simulink model "SkywalkerX8_Longitudinal_Control_Digital_Verification"  (R2018a)
settings: Solver=FixedStepAuto  StartTime=0.0  StopTime=10  RelTol=1e-3
undefined symbols (not defined in the file): DiscIntNeverNeededParam, SkywalkerX8
libraries: simulink_extras x5, simulink x1
settings Model: SnapshotInterval=1  Creator=David  LastModifiedBy=David
settings SolverCC: AlgebraicLoopSolver=LineSearch

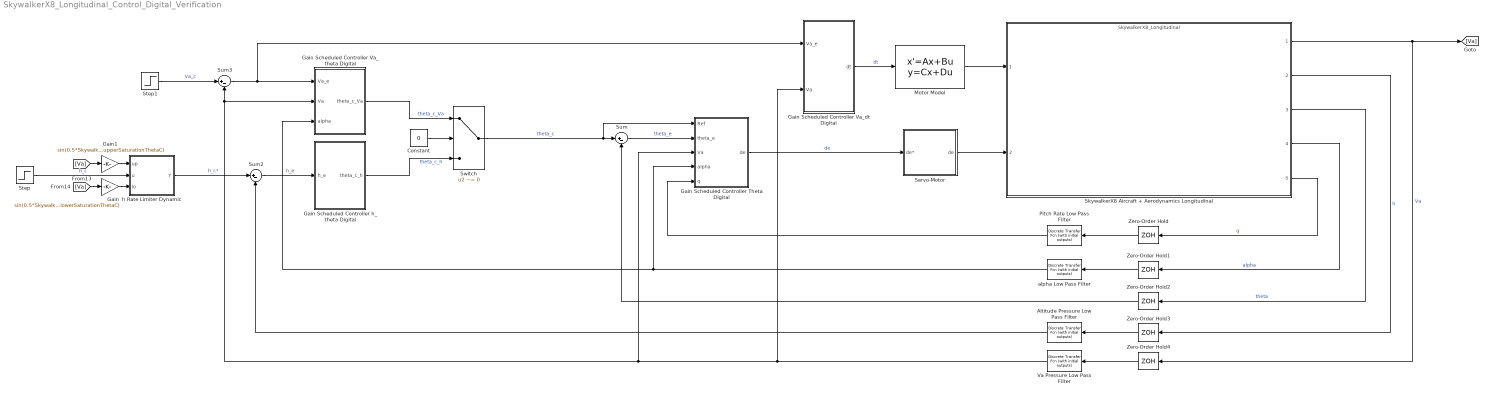
== system SkywalkerX8_Longitudinal_Control_Digital_Verification ==
  Altitude Pressure Low Pass Filter : simulink_extras/Additional Discrete/Discrete Transfer Fcn (with initial outputs)  N=cell2mat(SkywalkerX8.Sensors.Filters.AltitudePressure.FilterTFDigital.Numerator)  D=cell2mat(SkywalkerX8.Sensors.Filters.AltitudePressure.FilterTFDigital.Denominator)  U0=-SkywalkerX8.InitialConditions.XeYeZe(3)  Y0=-SkywalkerX8.InitialConditions.XeYeZe(3)  TS=SkywalkerX8.Sensors.Filters.AltitudePressure.FilterSampleTime
      settings: SourceProductName=Simulink  SourceProductBaseCode=SL
  Constant : Constant  Value=0  OutDataTypeStr=boolean
  Gain : Gain  Gain=sin(0.5*SkywalkerX8.Control.Longitudinal.altController.lowerSaturationThetaC)
  Gain Scheduled Controller Theta Digital : Subsystem
  Gain Scheduled Controller Va_dt Digital : Subsystem
  Gain Scheduled Controller Va_theta Digital : Subsystem
  Gain Scheduled Controller h_theta Digital : Subsystem
  Gain1 : Gain  Gain=sin(0.5*SkywalkerX8.Control.Longitudinal.altController.upperSaturationThetaC)
  Motor Model : StateSpace  A=SkywalkerX8.Actuators.Motor.SS.A  B=SkywalkerX8.Actuators.Motor.SS.B  C=SkywalkerX8.Actuators.Motor.SS.C  D=SkywalkerX8.Actuators.Motor.SS.D  InitialCondition=SkywalkerX8.InitialConditions.dt/SkywalkerX8.Actuators.Motor.SS.C
      mask Display: image('motor.jpg', 'center')
  Pitch Rate Low Pass Filter : simulink_extras/Additional Discrete/Discrete Transfer Fcn (with initial outputs)  N=cell2mat(SkywalkerX8.Sensors.Filters.AngularRates.Pitch.FilterTFDigital.Numerator)  D=cell2mat(SkywalkerX8.Sensors.Filters.AngularRates.Pitch.FilterTFDigital.Denominator)  U0=SkywalkerX8.Sensors.Filters.AngularRates.Pitch.InitialCondition  Y0=SkywalkerX8.Sensors.Filters.AngularRates.Pitch.InitialCondition  TS=SkywalkerX8.Sensors.Filters.AngularRates.Pitch.FilterSampleTime
      settings: SourceProductName=Simulink  SourceProductBaseCode=SL
  Servo-Motor : Subsystem
      mask Display: image('servo.jpg', 'center')
  SkywalkerX8 Aircraft + Aerodynamics Longitudinal : ModelReference  ModelNameDialog=SkywalkerX8_Longitudinal  ModelReferenceVersion=1.65
      mask Display:
      | image('x8SkySunset.png', 'center')
      | 
      | port_label('input', 1, '\delta_t (Unitless)', 'texmode', 'on')
      | port_label('input', 2, '\delta_e (rad)', 'texmode', 'on')
      | 
      | port_label('output', 1, 'V_a (m/s)', 'texmode', 'on')
      | port_label('output', 2, 'Altitude (m)', 'texmode', 'on')
      | port_label('output', 3, '\theta (rad)', 'texmode', 'on')
      | port_label('output', 4, 'alpha (rad)', 'texmode', 'on')
      | port_label('output', 5, 'q (rad/s)', 'texmode', 'on')
  Step : Step  Time=0.1  Before=-SkywalkerX8.InitialConditions.XeYeZe(3)  After=-SkywalkerX8.InitialConditions.XeYeZe(3)  SampleTime=0
  Step1 : Step  Time=5  Before=sqrt(SkywalkerX8.InitialConditions.uvw*SkywalkerX8.InitialConditions.uvw')  After=1.25*sqrt(SkywalkerX8.InitialConditions.uvw*SkywalkerX8.InitialConditions.uvw')  SampleTime=0
  Sum : Sum  Inputs=|+-
  Sum2 : Sum  Inputs=|+-
  Sum3 : Sum  Inputs=|+-
  Switch : Switch  Criteria=u2 ~= 0
  Va Pressure Low Pass Filter : simulink_extras/Additional Discrete/Discrete Transfer Fcn (with initial outputs)  N=cell2mat(SkywalkerX8.Sensors.Filters.AirspeedPressure.FilterTFDigital.Numerator)  D=cell2mat(SkywalkerX8.Sensors.Filters.AirspeedPressure.FilterTFDigital.Denominator)  U0=sqrt(SkywalkerX8.InitialConditions.uvw*SkywalkerX8.InitialConditions.uvw')  Y0=sqrt(SkywalkerX8.InitialConditions.uvw*SkywalkerX8.InitialConditions.uvw')  TS=SkywalkerX8.Sensors.Filters.AirspeedPressure.FilterSampleTime
      settings: SourceProductName=Simulink  SourceProductBaseCode=SL
  Zero-Order Hold : ZeroOrderHold  SampleTime=SkywalkerX8.Sensors.IMU.Gyroscope.SampleTime
  Zero-Order Hold1 : ZeroOrderHold  SampleTime=SkywalkerX8.Sensors.AoA.SampleTime
  Zero-Order Hold2 : ZeroOrderHold  SampleTime=SkywalkerX8.Sensors.EKF.GPSSmoothing.StateTransitionSampleTime
  Zero-Order Hold3 : ZeroOrderHold  SampleTime=SkywalkerX8.Sensors.AltitudePressure.SampleTime
  Zero-Order Hold4 : ZeroOrderHold  SampleTime=SkywalkerX8.Sensors.AirspeedPressure.SampleTime
  alpha Low Pass Filter : simulink_extras/Additional Discrete/Discrete Transfer Fcn (with initial outputs)  N=cell2mat(SkywalkerX8.Sensors.Filters.AoA.FilterTFDigital.Numerator)  D=cell2mat(SkywalkerX8.Sensors.Filters.AoA.FilterTFDigital.Denominator)  U0=SkywalkerX8.Sensors.Filters.AoA.InitialCondition  Y0=SkywalkerX8.Sensors.Filters.AoA.InitialCondition  TS=SkywalkerX8.Sensors.Filters.AoA.FilterSampleTime
      settings: SourceProductName=Simulink  SourceProductBaseCode=SL
  h Rate Limiter Dynamic : Subsystem  mask{initOutput=-SkywalkerX8.InitialConditions.XeYeZe(3)}
      mask prompts: initOutput "Initial output of dynamic rate limiter"
      mask DialogControl DescGroupVar Prompt: Rate Limiter Dynamic
      mask DialogControl DescTextVar Prompt: Limit rising and falling rates of the signals at the second input by using the first input (upper limit) and the third input (lower limit).
      mask Display:
      | image('rateLimit.png')
      | 
      | port_label('input', 1, 'up')
      | port_label('input', 2, 'u')
      | port_label('input', 3, 'lo')
      | 
      | port_label('output', 1, 'Y')
  wires:
  SkywalkerX8 Aircraft + Aerodynamics Longitudinal/5 -> Zero-Order Hold/1  "q"
  SkywalkerX8 Aircraft + Aerodynamics Longitudinal/3 -> Zero-Order Hold2/1  "theta"
  Constant/1 -> Switch/2
  SkywalkerX8 Aircraft + Aerodynamics Longitudinal/2 -> Zero-Order Hold3/1  "h"
  Sum2/1 -> Gain Scheduled Controller h_theta Digital/1(h_e)  "h_e"
  SkywalkerX8 Aircraft + Aerodynamics Longitudinal/1 -> Zero-Order Hold4/1, [Va]  "Va"
  Gain Scheduled Controller Va_theta Digital/1(theta_c_Va) -> Switch/1  "theta_c_Va"
  Step1/1 -> Sum3/1  "Va_c"
  Sum/1 -> Gain Scheduled Controller Theta Digital/2(theta_e)  "theta_e"
  SkywalkerX8 Aircraft + Aerodynamics Longitudinal/4 -> Zero-Order Hold1/1  "alpha"
  Gain Scheduled Controller h_theta Digital/1(theta_c_h) -> Switch/3  "theta_c_h"
  Gain Scheduled Controller Va_dt Digital/1(dt) -> Motor Model/1  "dt"
  h Rate Limiter Dynamic/1(Y) -> Sum2/1  "h_c*"
  Gain Scheduled Controller Theta Digital/1(de) -> Servo-Motor/1(de*)  "de"
  Sum3/1 -> Gain Scheduled Controller Va_theta Digital/1(Va_e), Gain Scheduled Controller Va_dt Digital/1(Va_e)
  Zero-Order Hold1/1 -> alpha Low Pass Filter/1
  Zero-Order Hold3/1 -> Altitude Pressure Low Pass Filter/1
  Zero-Order Hold4/1 -> Va Pressure Low Pass Filter/1
  Motor Model/1 -> SkywalkerX8 Aircraft + Aerodynamics Longitudinal/1
  Servo-Motor/1(de) -> SkywalkerX8 Aircraft + Aerodynamics Longitudinal/2
  Switch/1 -> Gain Scheduled Controller Theta Digital/1(Ref), Sum/1  "theta_c"
  Gain/1 -> h Rate Limiter Dynamic/3(lo)
  [Va] -> Gain1/1
  Gain1/1 -> h Rate Limiter Dynamic/1(up)
  [Va] -> Gain/1
  Step/1 -> h Rate Limiter Dynamic/2(u)  "h_c"
  Zero-Order Hold2/1 -> Sum/2
  Zero-Order Hold/1 -> Pitch Rate Low Pass Filter/1
  Altitude Pressure Low Pass Filter/1 -> Sum2/2
  Va Pressure Low Pass Filter/1 -> Gain Scheduled Controller Va_theta Digital/2(Va), Sum3/2, Gain Scheduled Controller Theta Digital/3(Va), Gain Scheduled Controller Va_dt Digital/2(Va)
  Pitch Rate Low Pass Filter/1 -> Gain Scheduled Controller Theta Digital/5(q)
  alpha Low Pass Filter/1 -> Gain Scheduled Controller Theta Digital/4(alpha), Gain Scheduled Controller Va_theta Digital/3(alpha)

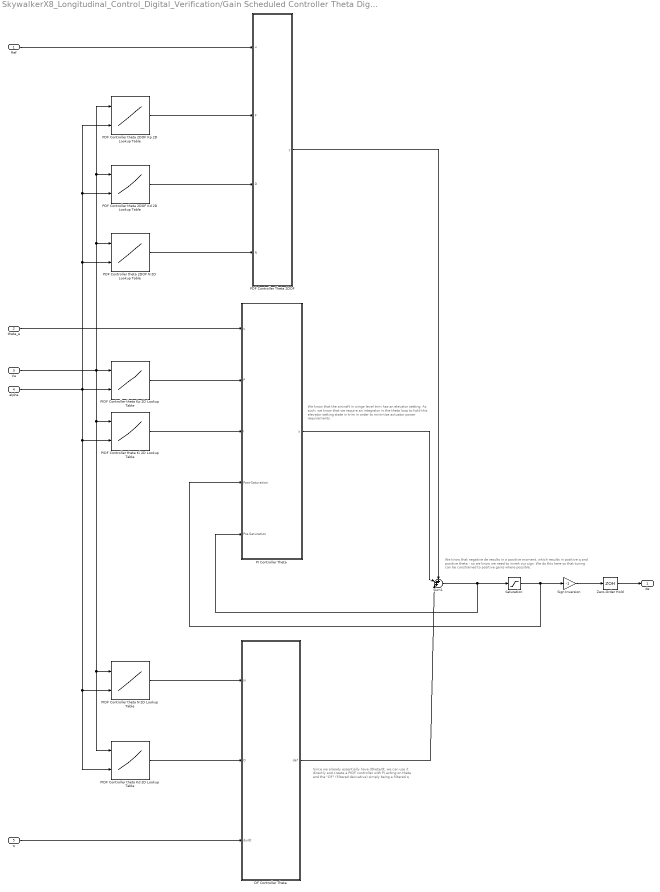
== system SkywalkerX8_Longitudinal_Control_Digital_Verification/Gain Scheduled Controller Theta Digital ==
  note: Since we already essentially have dtheta/dt,
      | we can use it directly and create a PIDF controller
      | with PI acting on theta and the "DF" (filtered derivative)
      | simply being a filtered q
  note: We know that negative de results in a positive moment, which results in
      | positive q and positive theta - so we know we need to invert our sign.
      | We do this here so that tuning can be constrained to positive gains where possible.
  note: We know that the aircraft in wings-level trim has an elevator setting. As such, we know that we require an integrator in the theta loop to hold this elevator setting state in trim in order to minimize actuator power requirements.
  Ref : Inport
  theta_e : Inport  Port=2
  Va : Inport  Port=3
  alpha : Inport  Port=4
  q : Inport  Port=5
  DF Controller Theta : Subsystem
  PDF Controller Theta 2DOF : Subsystem
  PDF Controller theta 2DOF Kd 2D Lookup Table : Lookup_n-D  BreakpointsForDimension1=SkywalkerX8.Control.Longitudinal.SchedulingVariables.VaArray  BreakpointsForDimension2=SkywalkerX8.Control.Longitudinal.SchedulingVariables.alphaArray  Table=SkywalkerX8.Control.Longitudinal.thetaController.Digital.KdTheta2DOF  InternalRulePriority=Speed  RndMeth=Simplest  InputSameDT=on
  PDF Controller theta 2DOF Kp 2D Lookup Table : Lookup_n-D  BreakpointsForDimension1=SkywalkerX8.Control.Longitudinal.SchedulingVariables.VaArray  BreakpointsForDimension2=SkywalkerX8.Control.Longitudinal.SchedulingVariables.alphaArray  Table=SkywalkerX8.Control.Longitudinal.thetaController.Digital.KpTheta2DOF  InternalRulePriority=Speed  RndMeth=Simplest  InputSameDT=on
  PDF Controller theta 2DOF N 2D Lookup Table : Lookup_n-D  BreakpointsForDimension1=SkywalkerX8.Control.Longitudinal.SchedulingVariables.VaArray  BreakpointsForDimension2=SkywalkerX8.Control.Longitudinal.SchedulingVariables.alphaArray  Table=SkywalkerX8.Control.Longitudinal.thetaController.Digital.NTheta2DOF  InternalRulePriority=Speed  RndMeth=Simplest  InputSameDT=on
  PI Controller Theta : Subsystem
  PIDF Controller theta Kd 2D Lookup Table : Lookup_n-D  BreakpointsForDimension1=SkywalkerX8.Control.Longitudinal.SchedulingVariables.VaArray  BreakpointsForDimension2=SkywalkerX8.Control.Longitudinal.SchedulingVariables.alphaArray  Table=SkywalkerX8.Control.Longitudinal.thetaController.Digital.KdTheta  InternalRulePriority=Speed  RndMeth=Simplest  InputSameDT=on
  PIDF Controller theta Ki 2D Lookup Table : Lookup_n-D  BreakpointsForDimension1=SkywalkerX8.Control.Longitudinal.SchedulingVariables.VaArray  BreakpointsForDimension2=SkywalkerX8.Control.Longitudinal.SchedulingVariables.alphaArray  Table=SkywalkerX8.Control.Longitudinal.thetaController.Digital.KiTheta  InternalRulePriority=Speed  RndMeth=Simplest  InputSameDT=on
  PIDF Controller theta Kp 2D Lookup Table : Lookup_n-D  BreakpointsForDimension1=SkywalkerX8.Control.Longitudinal.SchedulingVariables.VaArray  BreakpointsForDimension2=SkywalkerX8.Control.Longitudinal.SchedulingVariables.alphaArray  Table=SkywalkerX8.Control.Longitudinal.thetaController.Digital.KpTheta  InternalRulePriority=Speed  RndMeth=Simplest  InputSameDT=on
  PIDF Controller theta N 2D Lookup Table : Lookup_n-D  BreakpointsForDimension1=SkywalkerX8.Control.Longitudinal.SchedulingVariables.VaArray  BreakpointsForDimension2=SkywalkerX8.Control.Longitudinal.SchedulingVariables.alphaArray  Table=SkywalkerX8.Control.Longitudinal.thetaController.Digital.NTheta  InternalRulePriority=Speed  RndMeth=Simplest  InputSameDT=on
  Saturation : Saturate  UpperLimit=SkywalkerX8.Control.Longitudinal.thetaController.Digital.upperSaturationNegativeDe  LowerLimit=SkywalkerX8.Control.Longitudinal.thetaController.Digital.lowerSaturationNegativeDe
  Sign Inversion : Gain  Gain=-1
  Sum1 : Sum  Inputs=+++|
  Zero-Order Hold : ZeroOrderHold  SampleTime=SkywalkerX8.Control.Longitudinal.thetaController.Digital.SampleTime
  de : Outport
  wires:
  Va/1 -> PDF Controller theta 2DOF Kd 2D Lookup Table/1, PDF Controller theta 2DOF Kp 2D Lookup Table/1, PDF Controller theta 2DOF N 2D Lookup Table/1, PIDF Controller theta N 2D Lookup Table/1, PIDF Controller theta Kd 2D Lookup Table/1, PIDF Controller theta Ki 2D Lookup Table/1, PIDF Controller theta Kp 2D Lookup Table/1
  theta_e/1 -> PI Controller Theta/1(u)
  PIDF Controller theta Kp 2D Lookup Table/1 -> PI Controller Theta/2(P)
  PIDF Controller theta Ki 2D Lookup Table/1 -> PI Controller Theta/3(I)
  alpha/1 -> PDF Controller theta 2DOF N 2D Lookup Table/2, PDF Controller theta 2DOF Kd 2D Lookup Table/2, PDF Controller theta 2DOF Kp 2D Lookup Table/2, PIDF Controller theta N 2D Lookup Table/2, PIDF Controller theta Kd 2D Lookup Table/2, PIDF Controller theta Ki 2D Lookup Table/2, PIDF Controller theta Kp 2D Lookup Table/2
  PI Controller Theta/1(y) -> Sum1/2
  Sum1/1 -> Saturation/1, PI Controller Theta/5(Pre-Saturation)
  Saturation/1 -> Sign Inversion/1, PI Controller Theta/4(Post-Saturation)
  PIDF Controller theta N 2D Lookup Table/1 -> DF Controller Theta/1(N)
  PIDF Controller theta Kd 2D Lookup Table/1 -> DF Controller Theta/2(D)
  q/1 -> DF Controller Theta/3(du/dt)
  DF Controller Theta/1(de*) -> Sum1/3
  Sign Inversion/1 -> Zero-Order Hold/1
  PDF Controller theta 2DOF Kp 2D Lookup Table/1 -> PDF Controller Theta 2DOF/2(P)
  PDF Controller theta 2DOF Kd 2D Lookup Table/1 -> PDF Controller Theta 2DOF/3(D)
  PDF Controller theta 2DOF N 2D Lookup Table/1 -> PDF Controller Theta 2DOF/4(N)
  Ref/1 -> PDF Controller Theta 2DOF/1(u)
  PDF Controller Theta 2DOF/1(y) -> Sum1/1
  Zero-Order Hold/1 -> de/1

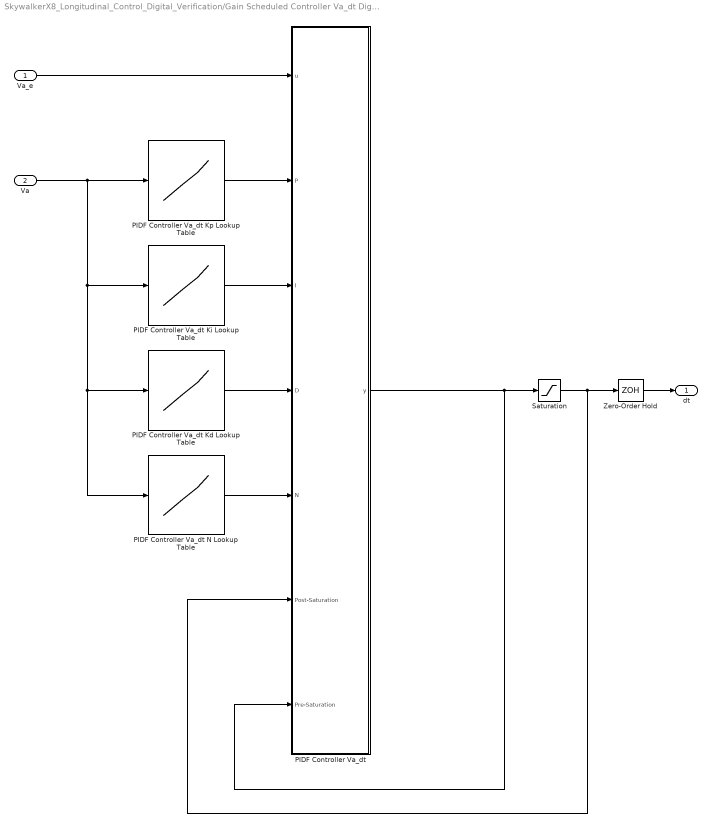
== system SkywalkerX8_Longitudinal_Control_Digital_Verification/Gain Scheduled Controller Va_dt Digital ==
  Va_e : Inport
  Va : Inport  Port=2
  PIDF Controller Va_dt : Subsystem
  PIDF Controller Va_dt Kd Lookup Table : Lookup_n-D  NumberOfTableDimensions=1  BreakpointsForDimension1=SkywalkerX8.Control.Longitudinal.SchedulingVariables.VaArray  BreakpointsForDimension2=[1 2 3 4 5]  Table=SkywalkerX8.Control.Longitudinal.VaDtController.Digital.KdVaDt  InternalRulePriority=Speed  RndMeth=Simplest  InputSameDT=on
  PIDF Controller Va_dt Ki Lookup Table : Lookup_n-D  NumberOfTableDimensions=1  BreakpointsForDimension1=SkywalkerX8.Control.Longitudinal.SchedulingVariables.VaArray  BreakpointsForDimension2=[1 2 3 4 5]  Table=SkywalkerX8.Control.Longitudinal.VaDtController.Digital.KiVaDt  InternalRulePriority=Speed  RndMeth=Simplest  InputSameDT=on
  PIDF Controller Va_dt Kp Lookup Table : Lookup_n-D  NumberOfTableDimensions=1  BreakpointsForDimension1=SkywalkerX8.Control.Longitudinal.SchedulingVariables.VaArray  BreakpointsForDimension2=[1 2 3 4 5]  Table=SkywalkerX8.Control.Longitudinal.VaDtController.Digital.KpVaDt  InternalRulePriority=Speed  RndMeth=Simplest  InputSameDT=on
  PIDF Controller Va_dt N Lookup Table : Lookup_n-D  NumberOfTableDimensions=1  BreakpointsForDimension1=SkywalkerX8.Control.Longitudinal.SchedulingVariables.VaArray  BreakpointsForDimension2=[1 2 3 4 5]  Table=SkywalkerX8.Control.Longitudinal.VaDtController.Digital.NVaDt  InternalRulePriority=Speed  RndMeth=Simplest  InputSameDT=on
  Saturation : Saturate  UpperLimit=SkywalkerX8.Control.Longitudinal.VaDtController.upperSaturationDt  LowerLimit=SkywalkerX8.Control.Longitudinal.VaDtController.lowerSaturationDt
  Zero-Order Hold : ZeroOrderHold  SampleTime=SkywalkerX8.Control.Longitudinal.VaDtController.Digital.SampleTime
  dt : Outport
  wires:
  Va_e/1 -> PIDF Controller Va_dt/1(u)
  Saturation/1 -> PIDF Controller Va_dt/6(Post-Saturation), Zero-Order Hold/1
  PIDF Controller Va_dt Kp Lookup Table/1 -> PIDF Controller Va_dt/2(P)
  Va/1 -> PIDF Controller Va_dt Kp Lookup Table/1, PIDF Controller Va_dt N Lookup Table/1, PIDF Controller Va_dt Kd Lookup Table/1, PIDF Controller Va_dt Ki Lookup Table/1
  PIDF Controller Va_dt Ki Lookup Table/1 -> PIDF Controller Va_dt/3(I)
  PIDF Controller Va_dt Kd Lookup Table/1 -> PIDF Controller Va_dt/4(D)
  PIDF Controller Va_dt N Lookup Table/1 -> PIDF Controller Va_dt/5(N)
  PIDF Controller Va_dt/1(y) -> Saturation/1, PIDF Controller Va_dt/7(Pre-Saturation)
  Zero-Order Hold/1 -> dt/1

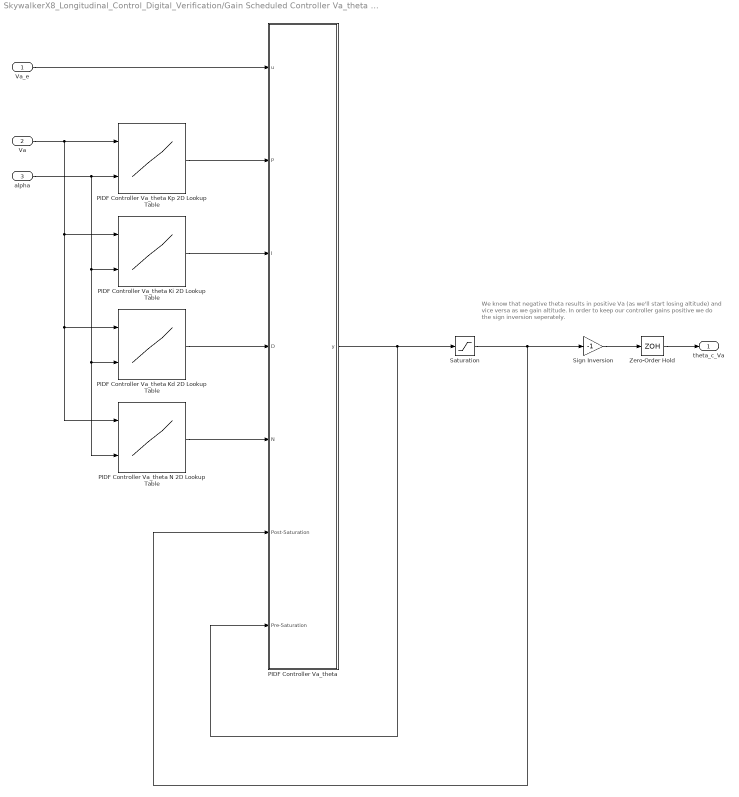
== system SkywalkerX8_Longitudinal_Control_Digital_Verification/Gain Scheduled Controller Va_theta Digital ==
  note: We know that negative theta results in positive Va (as we'll start losing altitude)
      | and vice versa as we gain altitude. In order to keep our controller gains positive
      |  we do the sign inversion seperately.
  Va_e : Inport
  Va : Inport  Port=2
  alpha : Inport  Port=3
  PIDF Controller Va_theta : Subsystem
  PIDF Controller Va_theta Kd 2D Lookup Table : Lookup_n-D  BreakpointsForDimension1=SkywalkerX8.Control.Longitudinal.SchedulingVariables.VaArray  BreakpointsForDimension2=SkywalkerX8.Control.Longitudinal.SchedulingVariables.alphaArray  Table=SkywalkerX8.Control.Longitudinal.VaThetaController.Digital.KdVaTheta  InternalRulePriority=Speed  RndMeth=Simplest  InputSameDT=on
  PIDF Controller Va_theta Ki 2D Lookup Table : Lookup_n-D  BreakpointsForDimension1=SkywalkerX8.Control.Longitudinal.SchedulingVariables.VaArray  BreakpointsForDimension2=SkywalkerX8.Control.Longitudinal.SchedulingVariables.alphaArray  Table=SkywalkerX8.Control.Longitudinal.VaThetaController.Digital.KiVaTheta  InternalRulePriority=Speed  RndMeth=Simplest  InputSameDT=on
  PIDF Controller Va_theta Kp 2D Lookup Table : Lookup_n-D  BreakpointsForDimension1=SkywalkerX8.Control.Longitudinal.SchedulingVariables.VaArray  BreakpointsForDimension2=SkywalkerX8.Control.Longitudinal.SchedulingVariables.alphaArray  Table=SkywalkerX8.Control.Longitudinal.VaThetaController.Digital.KpVaTheta  InternalRulePriority=Speed  RndMeth=Simplest  InputSameDT=on
  PIDF Controller Va_theta N 2D Lookup Table : Lookup_n-D  BreakpointsForDimension1=SkywalkerX8.Control.Longitudinal.SchedulingVariables.VaArray  BreakpointsForDimension2=SkywalkerX8.Control.Longitudinal.SchedulingVariables.alphaArray  Table=SkywalkerX8.Control.Longitudinal.VaThetaController.Digital.NVaTheta  InternalRulePriority=Speed  RndMeth=Simplest  InputSameDT=on
  Saturation : Saturate  UpperLimit=SkywalkerX8.Control.Longitudinal.VaThetaController.Digital.upperSaturationThetaC  LowerLimit=SkywalkerX8.Control.Longitudinal.VaThetaController.Digital.lowerSaturationThetaC
  Sign Inversion : Gain  Gain=-1
  Zero-Order Hold : ZeroOrderHold  SampleTime=SkywalkerX8.Control.Longitudinal.altController.Digital.SampleTime
  theta_c_Va : Outport
  wires:
  Va_e/1 -> PIDF Controller Va_theta/1(u)
  Saturation/1 -> Sign Inversion/1, PIDF Controller Va_theta/6(Post-Saturation)
  PIDF Controller Va_theta Kp 2D Lookup Table/1 -> PIDF Controller Va_theta/2(P)
  Va/1 -> PIDF Controller Va_theta Kd 2D Lookup Table/1, PIDF Controller Va_theta N 2D Lookup Table/1, PIDF Controller Va_theta Ki 2D Lookup Table/1, PIDF Controller Va_theta Kp 2D Lookup Table/1
  PIDF Controller Va_theta Ki 2D Lookup Table/1 -> PIDF Controller Va_theta/3(I)
  PIDF Controller Va_theta Kd 2D Lookup Table/1 -> PIDF Controller Va_theta/4(D)
  PIDF Controller Va_theta N 2D Lookup Table/1 -> PIDF Controller Va_theta/5(N)
  alpha/1 -> PIDF Controller Va_theta N 2D Lookup Table/2, PIDF Controller Va_theta Kd 2D Lookup Table/2, PIDF Controller Va_theta Ki 2D Lookup Table/2, PIDF Controller Va_theta Kp 2D Lookup Table/2
  Sign Inversion/1 -> Zero-Order Hold/1
  PIDF Controller Va_theta/1(y) -> Saturation/1, PIDF Controller Va_theta/7(Pre-Saturation)
  Zero-Order Hold/1 -> theta_c_Va/1

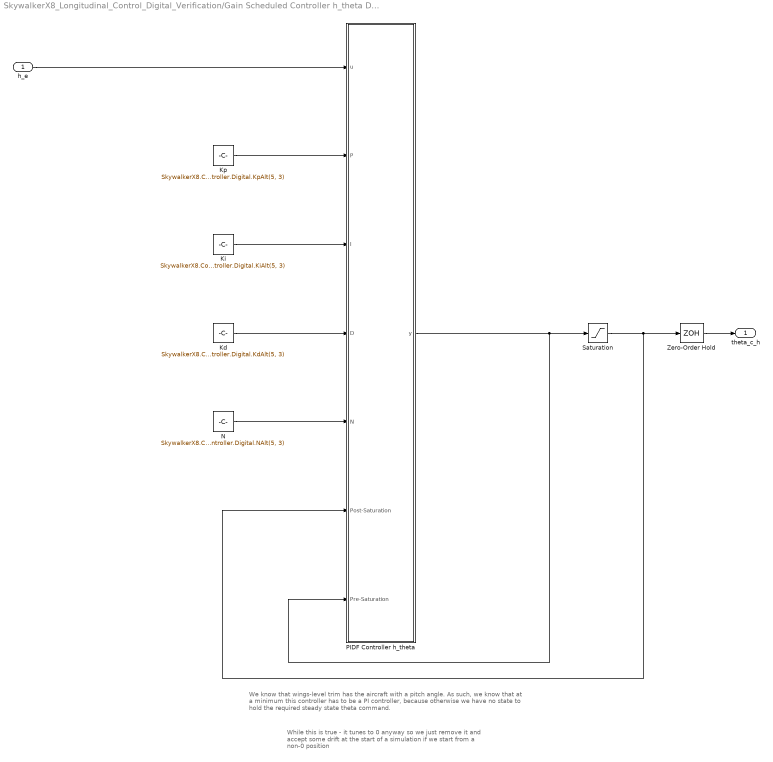
== system SkywalkerX8_Longitudinal_Control_Digital_Verification/Gain Scheduled Controller h_theta Digital ==
  note: While this is true - it tunes to 0 anyway so we just remove it
      | and accept some drift at the start of a simulation if we start
      | from a non-0 position
  note: We know that wings-level trim has the aircraft with a pitch angle. As such,
      | we know that at a minimum this controller has to be a PI controller, because otherwise
      | we have no state to hold the required steady state theta command.
  h_e : Inport
  Kd : Constant  Value=SkywalkerX8.Control.Longitudinal.altController.Digital.KdAlt(5, 3)
  Ki : Constant  Value=SkywalkerX8.Control.Longitudinal.altController.Digital.KiAlt(5, 3)
  Kp : Constant  Value=SkywalkerX8.Control.Longitudinal.altController.Digital.KpAlt(5, 3)
  N : Constant  Value=SkywalkerX8.Control.Longitudinal.altController.Digital.NAlt(5, 3)
  PIDF Controller h_theta : Subsystem
  Saturation : Saturate  UpperLimit=SkywalkerX8.Control.Longitudinal.altController.Digital.upperSaturationThetaC  LowerLimit=SkywalkerX8.Control.Longitudinal.altController.Digital.lowerSaturationThetaC
  Zero-Order Hold : ZeroOrderHold  SampleTime=SkywalkerX8.Control.Longitudinal.altController.Digital.SampleTime
  theta_c_h : Outport
  wires:
  Kp/1 -> PIDF Controller h_theta/2(P)
  h_e/1 -> PIDF Controller h_theta/1(u)
  Kd/1 -> PIDF Controller h_theta/4(D)
  N/1 -> PIDF Controller h_theta/5(N)
  Saturation/1 -> PIDF Controller h_theta/6(Post-Saturation), Zero-Order Hold/1
  PIDF Controller h_theta/1(y) -> PIDF Controller h_theta/7(Pre-Saturation), Saturation/1
  Ki/1 -> PIDF Controller h_theta/3(I)
  Zero-Order Hold/1 -> theta_c_h/1

== system SkywalkerX8_Longitudinal_Control_Digital_Verification/Servo-Motor ==
  de* : Inport
  Rate Limiter : RateLimiter  RisingSlewLimit=SkywalkerX8.Actuators.Servos.RateLimit  FallingSlewLimit=-SkywalkerX8.Actuators.Servos.RateLimit  SampleTimeMode=inherited  InitialCondition=SkywalkerX8.InitialConditions.de
  Saturation : Saturate  UpperLimit=2*SkywalkerX8.Actuators.Servos.UpperSaturation  LowerLimit=2*SkywalkerX8.Actuators.Servos.LowerSaturation
  Transfer Fcn (with initial outputs) : simulink_extras/Additional Linear/Transfer Fcn (with initial outputs)  N=cell2mat(SkywalkerX8.Actuators.Servos.TF.Numerator)  D=cell2mat(SkywalkerX8.Actuators.Servos.TF.Denominator)  Y0=SkywalkerX8.InitialConditions.de  U0=SkywalkerX8.InitialConditions.de
  de : Outport
  wires:
  Rate Limiter/1 -> Saturation/1
  de*/1 -> Transfer Fcn (with initial outputs)/1
  Saturation/1 -> de/1
  Transfer Fcn (with initial outputs)/1 -> Rate Limiter/1

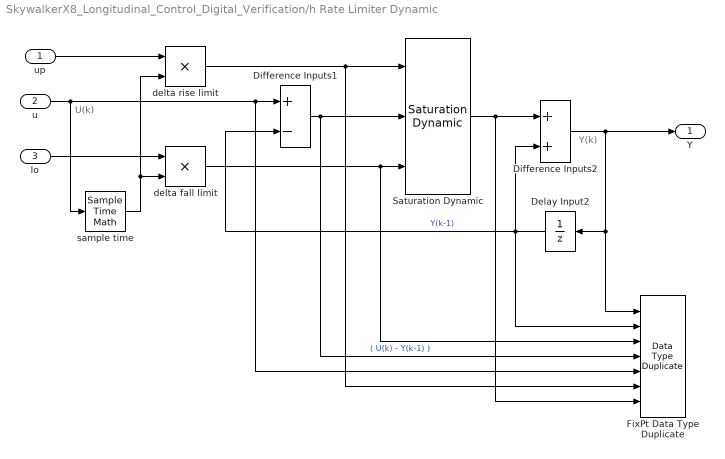
== system SkywalkerX8_Longitudinal_Control_Digital_Verification/h Rate Limiter Dynamic ==
  note: U(k)
  note: Y(k)
  up : Inport
  u : Inport  Port=2
  lo : Inport  Port=3
  Delay Input2 : UnitDelay  Description=Store in Global RAM  DisableCoverage=on  InitialCondition=initOutput  SampleTime=-1
  Difference Inputs1 : Sum  Description=Add in CPU  DisableCoverage=on  Inputs=+-  OutDataTypeStr=Inherit: Inherit via back propagation
  Difference Inputs2 : Sum  Description=Add in CPU  OutDataTypeStr=Inherit: Inherit via back propagation
  FixPt Data Type Duplicate : DataTypeDuplicate  DisableCoverage=on  NumInputPorts=7
  Saturation Dynamic : simulink/Discontinuities/Saturation Dynamic  OutMin=[]  OutMax=[]  OutDataTypeStr=Inherit: Same as second input  OutDataType=fixdt(1, 16)  OutScaling=2^-10  DoSatur=off
  delta fall limit : Product  DisableCoverage=on  Inputs=**  OutDataTypeStr=Inherit: Inherit via back propagation  SaturateOnIntegerOverflow=on
  delta rise limit : Product  DisableCoverage=on  Inputs=**  OutDataTypeStr=Inherit: Inherit via back propagation  SaturateOnIntegerOverflow=on
  sample time : SampleTimeMath  DisableCoverage=on  TsampMathOp=Ts Only  weightValue=1
  Y : Outport  InitialOutput=0
  wires:
  Delay Input2/1 -> Difference Inputs1/2, FixPt Data Type Duplicate/2, Difference Inputs2/2  "Y(k-1)"
  Difference Inputs1/1 -> FixPt Data Type Duplicate/4, Saturation Dynamic/2  "( U(k) - Y(k-1) )"
  Difference Inputs2/1 -> Y/1, Delay Input2/1, FixPt Data Type Duplicate/1
  u/1 -> Difference Inputs1/1, FixPt Data Type Duplicate/5, sample time/1
  delta fall limit/1 -> FixPt Data Type Duplicate/3, Saturation Dynamic/3
  sample time/1 -> delta fall limit/2, delta rise limit/2
  Saturation Dynamic/1 -> Difference Inputs2/1, FixPt Data Type Duplicate/7
  delta rise limit/1 -> FixPt Data Type Duplicate/6, Saturation Dynamic/1
  lo/1 -> delta fall limit/1
  up/1 -> delta rise limit/1

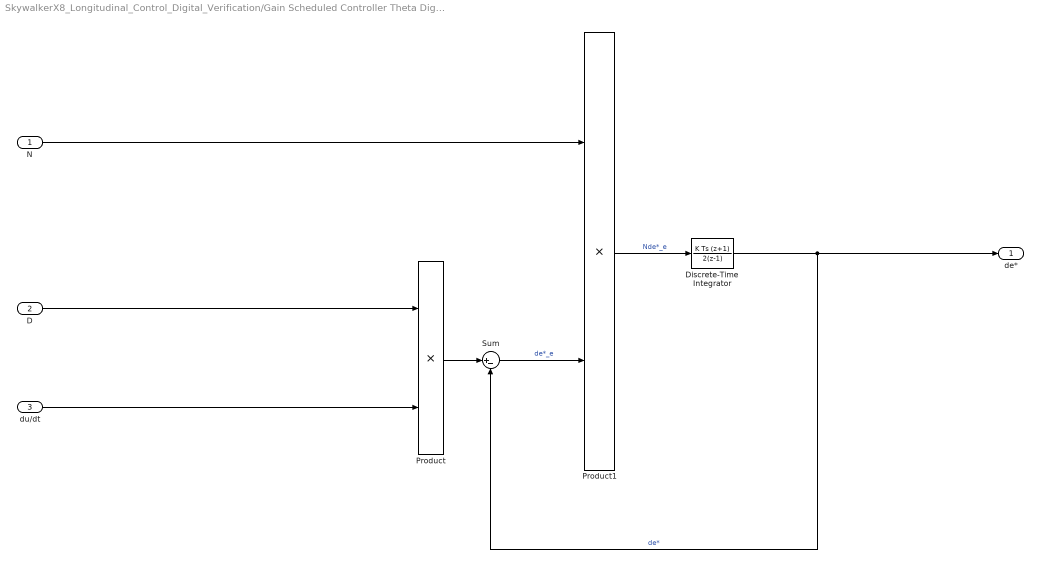
== system SkywalkerX8_Longitudinal_Control_Digital_Verification/Gain Scheduled Controller Theta Digital/DF Controller Theta ==
  N : Inport
  D : Inport  Port=2
  du/dt : Inport  Port=3
  Discrete-Time Integrator : DiscreteIntegrator  IntegratorMethod=Integration: Trapezoidal  SampleTime=SkywalkerX8.Control.Longitudinal.thetaController.Digital.SampleTime  ICPrevOutput=DiscIntNeverNeededParam  ICPrevScaledInput=DiscIntNeverNeededParam
  Product : Product
  Product1 : Product
  Sum : Sum  Inputs=|+-
  de* : Outport
  wires:
  Discrete-Time Integrator/1 -> de*/1, Sum/2  "de*"
  Product1/1 -> Discrete-Time Integrator/1  "Nde*_e"
  du/dt/1 -> Product/2
  D/1 -> Product/1
  Sum/1 -> Product1/2  "de*_e"
  N/1 -> Product1/1
  Product/1 -> Sum/1

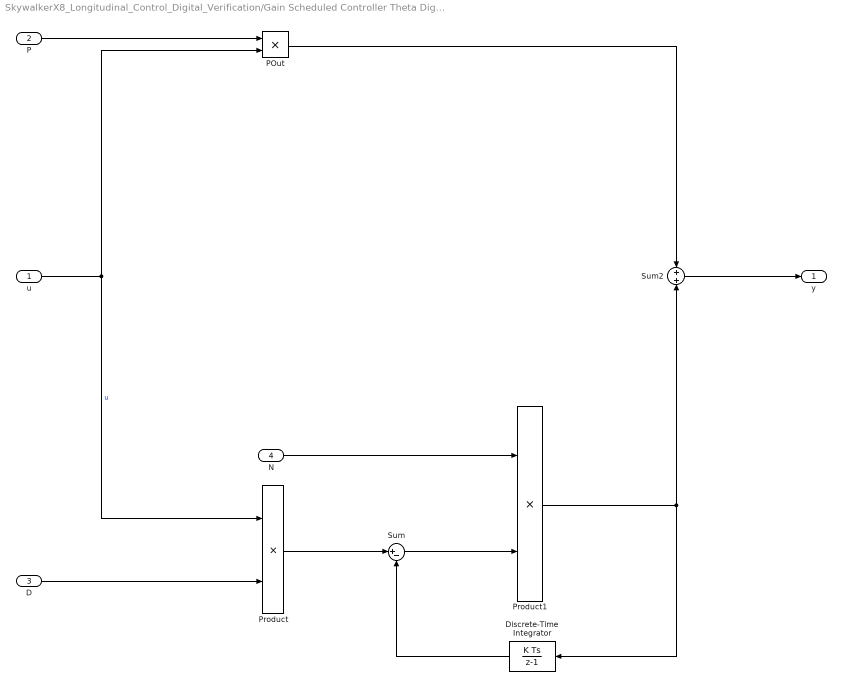
== system SkywalkerX8_Longitudinal_Control_Digital_Verification/Gain Scheduled Controller Theta Digital/PDF Controller Theta 2DOF ==
  u : Inport
  P : Inport  Port=2
  D : Inport  Port=3
  N : Inport  Port=4
  Discrete-Time Integrator : DiscreteIntegrator  SampleTime=SkywalkerX8.Control.Longitudinal.thetaController.Digital.SampleTime  ICPrevOutput=DiscIntNeverNeededParam  ICPrevScaledInput=DiscIntNeverNeededParam
  POut : Product
  Product : Product
  Product1 : Product
  Sum : Sum  Inputs=|+-
  Sum2 : Sum
  y : Outport  InitialOutput=0
  wires:
  Sum2/1 -> y/1
  N/1 -> Product1/1
  Product1/1 -> Discrete-Time Integrator/1, Sum2/2
  Sum/1 -> Product1/2
  POut/1 -> Sum2/1
  D/1 -> Product/2
  u/1 -> Product/1, POut/2  "u"
  Discrete-Time Integrator/1 -> Sum/2
  Product/1 -> Sum/1
  P/1 -> POut/1

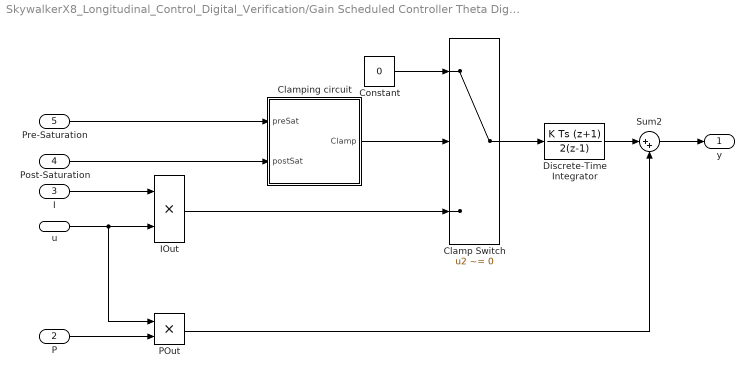
== system SkywalkerX8_Longitudinal_Control_Digital_Verification/Gain Scheduled Controller Theta Digital/PI Controller Theta ==
  u : Inport
  P : Inport  Port=2
  I : Inport  Port=3
  Post-Saturation : Inport  Port=4
  Pre-Saturation : Inport  Port=5
  Clamp Switch : Switch  Criteria=u2 ~= 0
  Clamping circuit : Subsystem
  Constant : Constant  Value=0
  Discrete-Time Integrator : DiscreteIntegrator  IntegratorMethod=Integration: Trapezoidal  InitialCondition=SkywalkerX8.InitialConditions.ThetaController.Integrator  SampleTime=SkywalkerX8.Control.Longitudinal.thetaController.Digital.SampleTime  ICPrevOutput=DiscIntNeverNeededParam  ICPrevScaledInput=DiscIntNeverNeededParam
  IOut : Product  DisableCoverage=on
  POut : Product
  Sum2 : Sum  Inputs=|++
  y : Outport  InitialOutput=0
  wires:
  IOut/1 -> Clamp Switch/3
  Clamp Switch/1 -> Discrete-Time Integrator/1
  Sum2/1 -> y/1
  Pre-Saturation/1 -> Clamping circuit/1(preSat)
  Post-Saturation/1 -> Clamping circuit/2(postSat)
  Clamping circuit/1(Clamp) -> Clamp Switch/2
  Constant/1 -> Clamp Switch/1
  Discrete-Time Integrator/1 -> Sum2/1
  POut/1 -> Sum2/2
  P/1 -> POut/2
  u/1 -> POut/1, IOut/2
  I/1 -> IOut/1

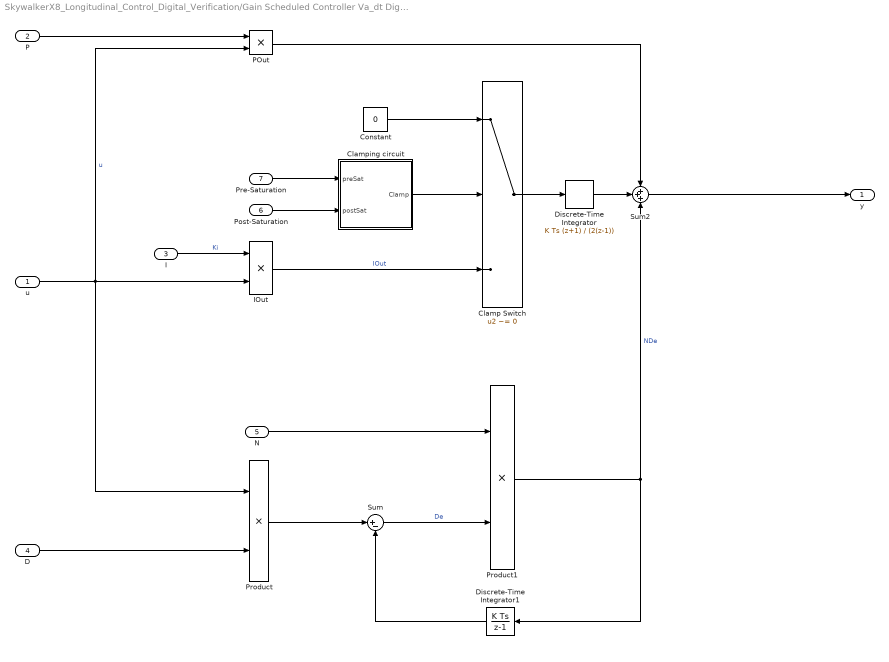
== system SkywalkerX8_Longitudinal_Control_Digital_Verification/Gain Scheduled Controller Va_dt Digital/PIDF Controller Va_dt ==
  u : Inport
  P : Inport  Port=2
  I : Inport  Port=3
  D : Inport  Port=4
  N : Inport  Port=5
  Post-Saturation : Inport  Port=6
  Pre-Saturation : Inport  Port=7
  Clamp Switch : Switch  Criteria=u2 ~= 0
  Clamping circuit : Subsystem
  Constant : Constant  Value=0
  Discrete-Time Integrator : DiscreteIntegrator  IntegratorMethod=Integration: Trapezoidal  InitialCondition=SkywalkerX8.InitialConditions.dt  SampleTime=SkywalkerX8.Control.Longitudinal.VaDtController.Digital.SampleTime  ICPrevOutput=DiscIntNeverNeededParam  ICPrevScaledInput=DiscIntNeverNeededParam
  Discrete-Time Integrator1 : DiscreteIntegrator  SampleTime=SkywalkerX8.Control.Longitudinal.VaDtController.Digital.SampleTime  ICPrevOutput=DiscIntNeverNeededParam  ICPrevScaledInput=DiscIntNeverNeededParam
  IOut : Product  DisableCoverage=on
  POut : Product
  Product : Product
  Product1 : Product
  Sum : Sum  Inputs=|+-
  Sum2 : Sum  Inputs=+++
  y : Outport  InitialOutput=0
  wires:
  Sum2/1 -> y/1
  N/1 -> Product1/1
  Product1/1 -> Discrete-Time Integrator1/1, Sum2/3  "NDe"
  Sum/1 -> Product1/2  "De"
  POut/1 -> Sum2/1
  D/1 -> Product/2
  u/1 -> POut/2, Product/1, IOut/2  "u"
  Discrete-Time Integrator1/1 -> Sum/2
  Clamp Switch/1 -> Discrete-Time Integrator/1
  Product/1 -> Sum/1
  Discrete-Time Integrator/1 -> Sum2/2
  Constant/1 -> Clamp Switch/1
  I/1 -> IOut/1  "Ki"
  IOut/1 -> Clamp Switch/3  "IOut"
  Clamping circuit/1(Clamp) -> Clamp Switch/2
  P/1 -> POut/1
  Pre-Saturation/1 -> Clamping circuit/1(preSat)
  Post-Saturation/1 -> Clamping circuit/2(postSat)

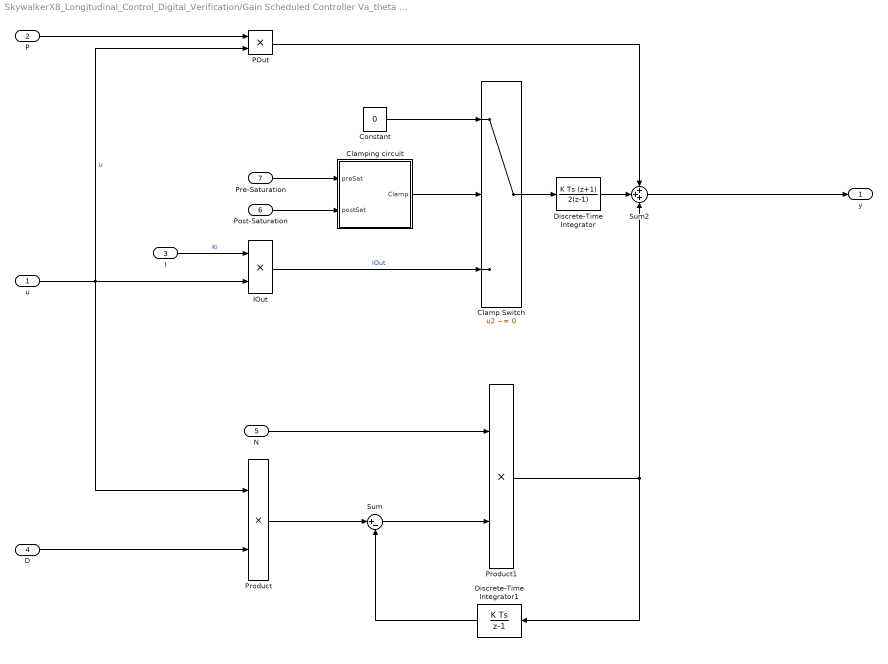
== system SkywalkerX8_Longitudinal_Control_Digital_Verification/Gain Scheduled Controller Va_theta Digital/PIDF Controller Va_theta ==
  u : Inport
  P : Inport  Port=2
  I : Inport  Port=3
  D : Inport  Port=4
  N : Inport  Port=5
  Post-Saturation : Inport  Port=6
  Pre-Saturation : Inport  Port=7
  Clamp Switch : Switch  Criteria=u2 ~= 0
  Clamping circuit : Subsystem
  Constant : Constant  Value=0
  Discrete-Time Integrator : DiscreteIntegrator  IntegratorMethod=Integration: Trapezoidal  InitialCondition=-SkywalkerX8.InitialConditions.PhiThetaPsi(2)  SampleTime=SkywalkerX8.Control.Longitudinal.VaThetaController.Digital.SampleTime  ICPrevOutput=DiscIntNeverNeededParam  ICPrevScaledInput=DiscIntNeverNeededParam
  Discrete-Time Integrator1 : DiscreteIntegrator  SampleTime=SkywalkerX8.Control.Longitudinal.VaThetaController.Digital.SampleTime  ICPrevOutput=DiscIntNeverNeededParam  ICPrevScaledInput=DiscIntNeverNeededParam
  IOut : Product  DisableCoverage=on
  POut : Product
  Product : Product
  Product1 : Product
  Sum : Sum  Inputs=|+-
  Sum2 : Sum  Inputs=+++
  y : Outport  InitialOutput=0
  wires:
  Sum2/1 -> y/1
  N/1 -> Product1/1
  Product1/1 -> Discrete-Time Integrator1/1, Sum2/3
  Sum/1 -> Product1/2
  POut/1 -> Sum2/1
  D/1 -> Product/2
  u/1 -> POut/2, Product/1, IOut/2  "u"
  Discrete-Time Integrator1/1 -> Sum/2
  Clamp Switch/1 -> Discrete-Time Integrator/1
  Product/1 -> Sum/1
  Discrete-Time Integrator/1 -> Sum2/2
  Constant/1 -> Clamp Switch/1
  I/1 -> IOut/1  "Ki"
  IOut/1 -> Clamp Switch/3  "IOut"
  Clamping circuit/1(Clamp) -> Clamp Switch/2
  P/1 -> POut/1
  Pre-Saturation/1 -> Clamping circuit/1(preSat)
  Post-Saturation/1 -> Clamping circuit/2(postSat)

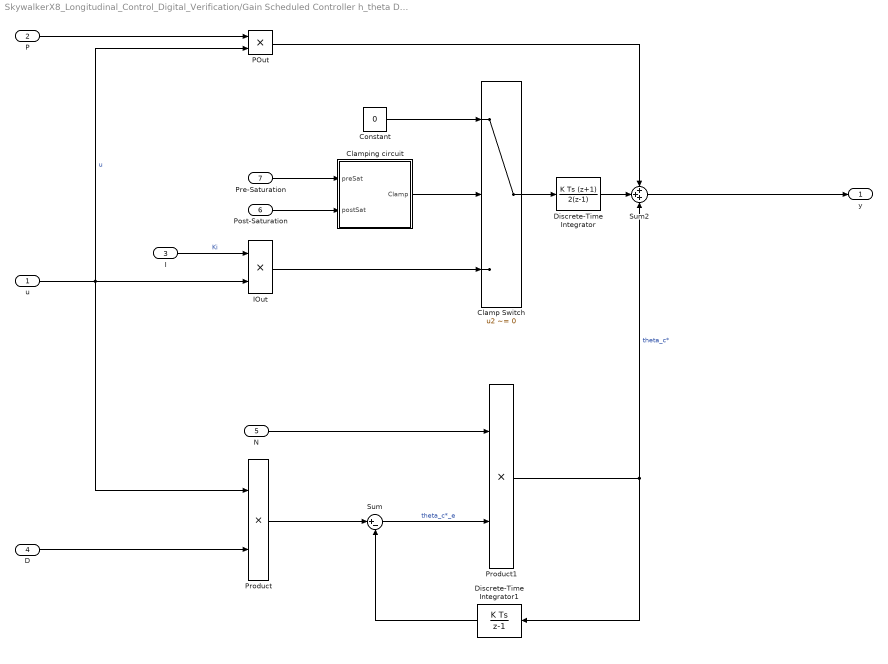
== system SkywalkerX8_Longitudinal_Control_Digital_Verification/Gain Scheduled Controller h_theta Digital/PIDF Controller h_theta ==
  u : Inport
  P : Inport  Port=2
  I : Inport  Port=3
  D : Inport  Port=4
  N : Inport  Port=5
  Post-Saturation : Inport  Port=6
  Pre-Saturation : Inport  Port=7
  Clamp Switch : Switch  Criteria=u2 ~= 0
  Clamping circuit : Subsystem
  Constant : Constant  Value=0
  Discrete-Time Integrator : DiscreteIntegrator  IntegratorMethod=Integration: Trapezoidal  InitialCondition=SkywalkerX8.InitialConditions.PhiThetaPsi(2)  SampleTime=SkywalkerX8.Control.Longitudinal.altController.Digital.SampleTime  ICPrevOutput=DiscIntNeverNeededParam  ICPrevScaledInput=DiscIntNeverNeededParam
  Discrete-Time Integrator1 : DiscreteIntegrator  SampleTime=SkywalkerX8.Control.Longitudinal.altController.Digital.SampleTime  ICPrevOutput=DiscIntNeverNeededParam  ICPrevScaledInput=DiscIntNeverNeededParam
  IOut : Product  DisableCoverage=on
  POut : Product
  Product : Product
  Product1 : Product
  Sum : Sum  Inputs=|+-
  Sum2 : Sum  Inputs=+++
  y : Outport  InitialOutput=0
  wires:
  Sum2/1 -> y/1
  N/1 -> Product1/1
  Product1/1 -> Sum2/3, Discrete-Time Integrator1/1  "theta_c*"
  Sum/1 -> Product1/2  "theta_c*_e"
  POut/1 -> Sum2/1
  D/1 -> Product/2
  u/1 -> POut/2, Product/1, IOut/2  "u"
  Discrete-Time Integrator1/1 -> Sum/2
  Clamp Switch/1 -> Discrete-Time Integrator/1
  Product/1 -> Sum/1
  Discrete-Time Integrator/1 -> Sum2/2
  Constant/1 -> Clamp Switch/1
  I/1 -> IOut/1  "Ki"
  IOut/1 -> Clamp Switch/3
  Clamping circuit/1(Clamp) -> Clamp Switch/2
  P/1 -> POut/1
  Pre-Saturation/1 -> Clamping circuit/1(preSat)
  Post-Saturation/1 -> Clamping circuit/2(postSat)

== system SkywalkerX8_Longitudinal_Control_Digital_Verification/Gain Scheduled Controller Theta Digital/PI Controller Theta/Clamping circuit ==
  preSat : Inport  DisableCoverage=on
  postSat : Inport  DisableCoverage=on  Port=2
  Memory : Memory  DisableCoverage=on
  NotEqual : RelationalOperator  DisableCoverage=on  Operator=~=  RndMeth=Nearest  InputSameDT=on
  Clamp : Outport  DisableCoverage=on
  wires:
  postSat/1 -> NotEqual/2
  preSat/1 -> NotEqual/1
  NotEqual/1 -> Memory/1
  Memory/1 -> Clamp/1

== system SkywalkerX8_Longitudinal_Control_Digital_Verification/Gain Scheduled Controller Va_dt Digital/PIDF Controller Va_dt/Clamping circuit ==
  preSat : Inport  DisableCoverage=on
  postSat : Inport  DisableCoverage=on  Port=2
  Memory : Memory  DisableCoverage=on
  NotEqual : RelationalOperator  DisableCoverage=on  Operator=~=  RndMeth=Nearest  InputSameDT=on
  Clamp : Outport  DisableCoverage=on
  wires:
  postSat/1 -> NotEqual/2
  preSat/1 -> NotEqual/1
  NotEqual/1 -> Memory/1
  Memory/1 -> Clamp/1

== system SkywalkerX8_Longitudinal_Control_Digital_Verification/Gain Scheduled Controller Va_theta Digital/PIDF Controller Va_theta/Clamping circuit ==
  preSat : Inport  DisableCoverage=on
  postSat : Inport  DisableCoverage=on  Port=2
  Memory : Memory  DisableCoverage=on
  NotEqual : RelationalOperator  DisableCoverage=on  Operator=~=  RndMeth=Nearest  InputSameDT=on
  Clamp : Outport  DisableCoverage=on
  wires:
  postSat/1 -> NotEqual/2
  preSat/1 -> NotEqual/1
  NotEqual/1 -> Memory/1
  Memory/1 -> Clamp/1

== system SkywalkerX8_Longitudinal_Control_Digital_Verification/Gain Scheduled Controller h_theta Digital/PIDF Controller h_theta/Clamping circuit ==
  preSat : Inport  DisableCoverage=on
  postSat : Inport  DisableCoverage=on  Port=2
  Memory : Memory  DisableCoverage=on
  NotEqual : RelationalOperator  DisableCoverage=on  Operator=~=  RndMeth=Nearest  InputSameDT=on
  Clamp : Outport  DisableCoverage=on
  wires:
  postSat/1 -> NotEqual/2
  preSat/1 -> NotEqual/1
  NotEqual/1 -> Memory/1
  Memory/1 -> Clamp/1
